simulink model "modal"  (R2022b)
settings: Solver=ode23tb  StartTime=0.0  StopTime=Tmdl  MaxStep=0.001  RelTol=1e-3
undefined symbols (not defined in the file or in its folder): k, modal
settings Model: Creator=osini  LastModifiedBy=osini

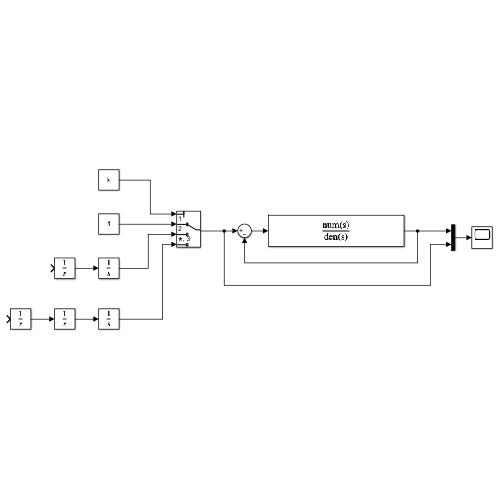
[thumbnail: Simulink's stored preview of the top-level diagram]
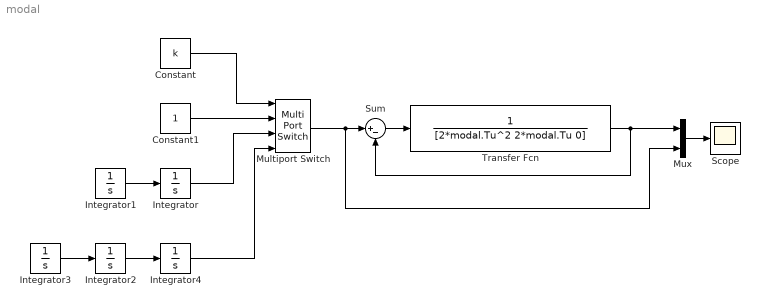
== system modal ==
  Constant : Constant  Value=k
  Constant1 : Constant
  Integrator : Integrator
  Integrator1 : Integrator  InitialCondition=1
  Integrator2 : Integrator
  Integrator3 : Integrator  InitialCondition=1
  Integrator4 : Integrator
  Multiport Switch : MultiPortSwitch  SaturateOnIntegerOverflow=off  InputSameDT=off
  Mux : Mux  Inputs=2
  Scope : Scope
  Sum : Sum  Inputs=|+-
  Transfer Fcn : TransferFcn  Denominator=[2*modal.Tu^2 2*modal.Tu 0]
  wires:
  Constant/1 -> Multiport Switch/1
  Mux/1 -> Scope/1
  Integrator4/1 -> Multiport Switch/4
  Integrator/1 -> Multiport Switch/3
  Multiport Switch/1 -> Mux/2, Sum/1
  Constant1/1 -> Multiport Switch/2
  Integrator1/1 -> Integrator/1
  Integrator2/1 -> Integrator4/1
  Integrator3/1 -> Integrator2/1
  Transfer Fcn/1 -> Mux/1, Sum/2
  Sum/1 -> Transfer Fcn/1
